simulink model "RC_circuit"  (R2020a)
settings: Solver=VariableStepAuto  StartTime=0.0  StopTime=50  MaxStep=0.001  RelTol=1e-3
PostLoadFcn:
  | R = 10;
  | C = 10*10^(-6);
settings Model: Creator=Admin  LastModifiedBy=Admin

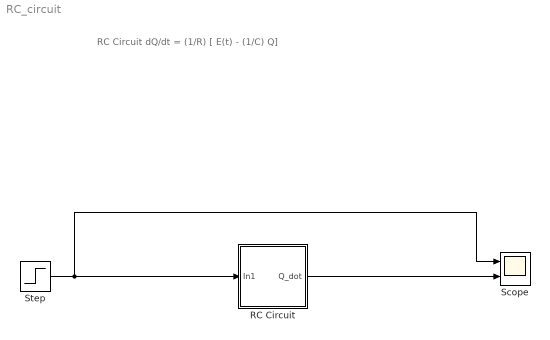
== system RC_circuit ==
  note: RC Circuit
      | dQ/dt = (1/R) [ E(t) - (1/C) Q]
  RC Circuit : Subsystem
  Scope : Scope  NumInputPorts=2
  Step : Step  SampleTime=0
  wires:
  Step/1 -> Scope/1, RC Circuit/1(In1)
  RC Circuit/1(Q_dot) -> Scope/2

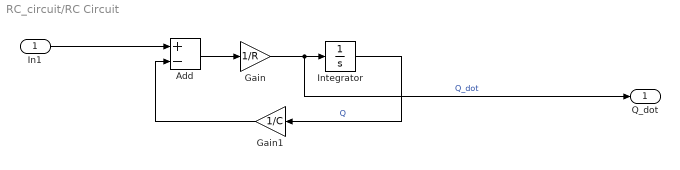
== system RC_circuit/RC Circuit ==
  In1 : Inport
  Add : Sum  Inputs=+-
  Gain : Gain  Gain=1/R
  Gain1 : Gain  Gain=1/C
  Integrator : Integrator
  Q_dot : Outport
  wires:
  Integrator/1 -> Gain1/1  "Q"
  Gain/1 -> Q_dot/1, Integrator/1  "Q_dot"
  Add/1 -> Gain/1
  Gain1/1 -> Add/2
  In1/1 -> Add/1
